simulink model "SerialSend"  (R2013a)
settings: Solver=ode45  StartTime=0.0  StopTime=inf  RelTol=1e-3
undefined symbols (not defined in the file or in its folder): none, Rec, SDTV, serial, videoinput
libraries: visionsinks x3, visionstatistics x2, imaqlib x2, instrumentlib x2, simulink x1, visionconversions x1, visiontextngfix x1, aerolibanimutils x1
settings Model: Creator=scastro  LastModifiedBy=sbiagion
settings OptimizationCC: ExpressionDepthLimit=2147483647  OptimizeModelRefInitCode=on  LifeSpan=1
settings DebuggingCC: StrictBusMsg=Warning
settings HardwareCC: ProdBitPerInt=16  ProdBitPerPointer=8  ProdIntDivRoundTo=Zero  ProdEndianess=LittleEndian  ProdWordSize=8  ProdHWDeviceType=Atmel->AVR
settings RTWCC: SystemTargetFile=realtime.tlc  GenerateMakefile=off  TemplateMakefile=realtime.tmf  Description=Real-Time Toolbox  RTWVerbose=off  ProcessScript=realtime_make_rtw_hook
settings CodeAppCC: IgnoreCustomStorageClasses=off  CustomSymbolStrType=$N$R$M  InternalIdentifier=Classic
settings STFCustomTargetCC: TargetLibSuffix=.a  GenerateSampleERTMain=on  CombineOutputUpdateFcns=on  ERTCustomFileBanners=on  SupportContinuousTime=off  SupportNonInlinedSFcns=off  MATLABClassNameForMDSCustomization=Simulink.SoftwareTarget.ERTCustomization  SystemTargetFile=realtime.tlc
settings ERTTargetCC: ParMdlRefBuildCompliant=off  CompOptLevelCompliant=off  ConcurrentExecutionCompliant=off  ERTFirstTimeCompliant=off  ModelStepFunctionPrototypeControlCompliant=off  CPPClassGenCompliant=off  ERTCustomFileTemplate=realtime_file_process.tlc

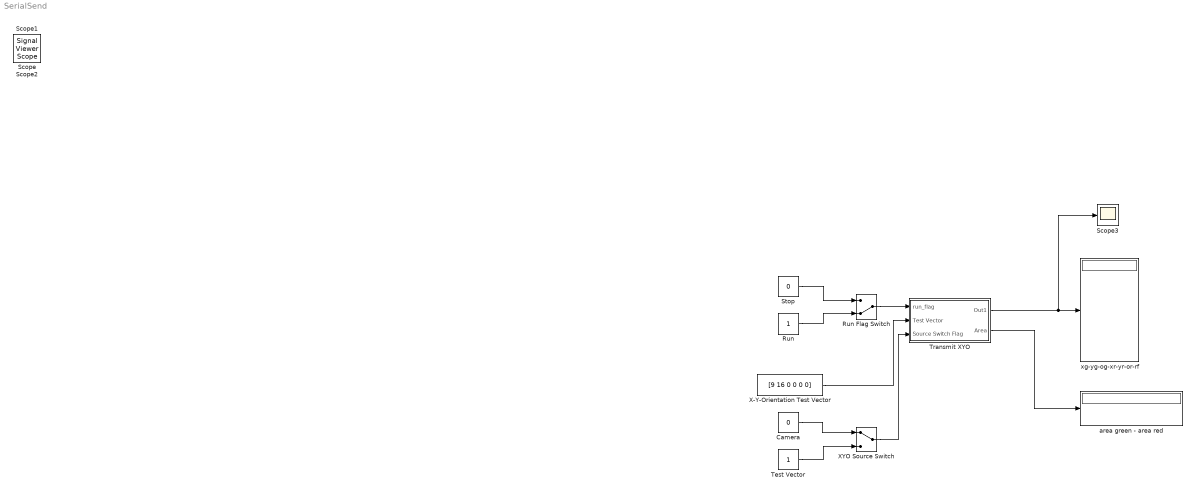
== system SerialSend ==
  Camera : Constant  Value=0  OutDataTypeStr=uint8
  Run : Constant  OutDataTypeStr=uint8
  Run Flag Switch : ManualSwitch  CurrentSetting=0
  Scope3 : Scope
      settings: ShowLegends=on  YMin=0  YMax=275
  Stop : Constant  Value=0  OutDataTypeStr=uint8
  Test Vector : Constant  OutDataTypeStr=uint8
  Transmit XYO : Subsystem
  X-Y-Orientation Test Vector : Constant  Value=[9 16 0 0 0 0]
  XYO Source Switch : ManualSwitch
  area green - area red : Display
  xg-yg-og-xr-yr-or-rf : Display
  Scope : SignalViewerScope  IOType=viewer  RefreshTime=0.035000
      settings: YMin=-40  YMax=70
  Scope1 : SignalViewerScope  IOType=viewer  ZoomMode=xonly  RefreshTime=0.035000
  Scope2 : SignalViewerScope  IOType=viewer  RefreshTime=0.035000
      settings: YMin=50  YMax=70  SaveName=ScopeData2
  wires:
  Run Flag Switch/1 -> Transmit XYO/1(run_flag)
  Stop/1 -> Run Flag Switch/1
  Run/1 -> Run Flag Switch/2
  Transmit XYO/1(Out1) -> Scope3/1, xg-yg-og-xr-yr-or-rf/1
  Camera/1 -> XYO Source Switch/1
  Test Vector/1 -> XYO Source Switch/2
  X-Y-Orientation Test Vector/1 -> Transmit XYO/2(Test Vector)
  XYO Source Switch/1 -> Transmit XYO/3(Source Switch Flag)
  Transmit XYO/2(Area) -> area green - area red/1

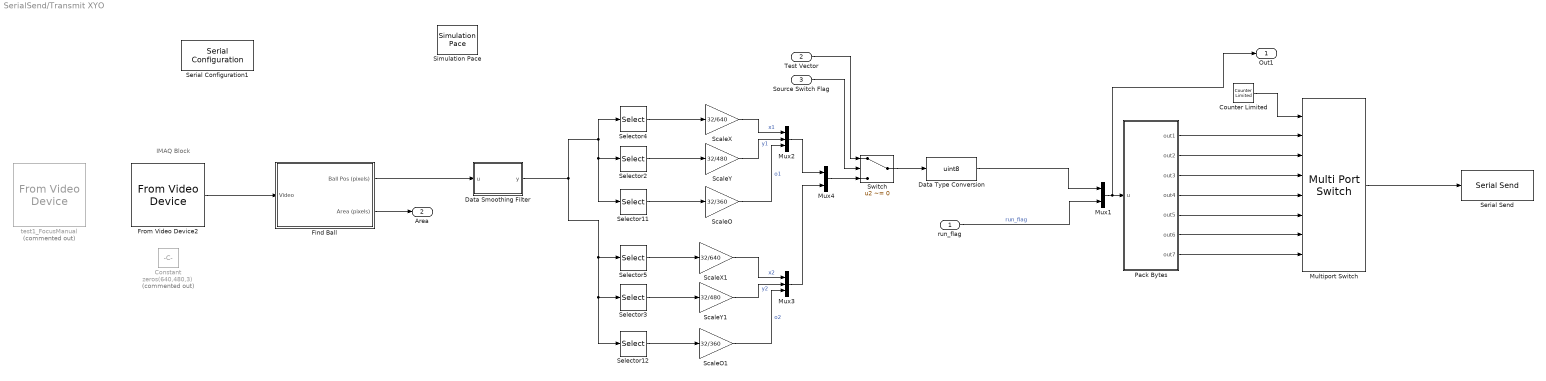
== system SerialSend/Transmit XYO ==
  note: IMAQ Block
  run_flag : Inport
  Test Vector : Inport  Port=2
  Source Switch Flag : Inport  Port=3
  Constant : Constant  Commented=on  Value=zeros(640,480,3)  SampleTime=0.1
  Counter Limited : simulink/Sources/Counter Limited  uplimit=6  tsamp=-1
  Data Smoothing Filter : MATLAB Function  TreatAsAtomicUnit=on
  Data Type Conversion : DataTypeConversion  OutDataTypeStr=uint8
  Find Ball : Subsystem
  From Video Device2 : imaqlib/From Video Device  DeviceMenu=winvideo 1 (Logitech Webcam Pro 9000)  Device=winvideo 1 (Logitech Webcam Pro 9000)  ObjConstructor=videoinput('winvideo', 1)  VideoFormatMenu=I420_640x480  VideoFormat=I420_640x480  VideoSource=input1  ROIPosition=[0 0 480 640]  EnableHWTrigger=off  TriggerConfiguration=none/none  SampleTime=0.1  OutputPortsMode=One multidimensional signal  DataType=double  CanDoHWTrigger=no  ReturnedColorSpace=rgb  BlockHandle=41.0012  ROIWidth=640  ROIHeight=480  ROIColumn=0  ROIRow=0  EngXMLPath=C:\Program Files\MATLAB\R2013a\toolbox\imaq\imaq\private  DevXMLPath=C:\Program Files\MATLAB\R2013a\toolbox\imaq\imaqadaptors\win64  EngLibPath=C:\Program Files\MATLAB\R2013a\toolbox\imaq\imaqblks\imaqmex\win64  ColorSpace=rgb  BayerSensorAlignment=grbg
  Multiport Switch : MultiPortSwitch  DataPortOrder=Zero-based contiguous  Inputs=7
  Mux1 : Mux  Inputs=2
  Mux2 : Mux  Inputs=3
  Mux3 : Mux  Inputs=3
  Mux4 : Mux  Inputs=2
  Pack Bytes : MATLAB Function  TreatAsAtomicUnit=on
  ScaleO : Gain  Gain=32/360
  ScaleO1 : Gain  Gain=32/360
  ScaleX : Gain  Gain=32/640
  ScaleX1 : Gain  Gain=32/640
  ScaleY : Gain  Gain=32/480
  ScaleY1 : Gain  Gain=32/480
  Selector11 : Selector  InputPortWidth=6  IndexOptions=Index vector (dialog)  Indices=3  OutputSizes=1
  Selector12 : Selector  InputPortWidth=6  IndexOptions=Index vector (dialog)  Indices=6  OutputSizes=1
  Selector2 : Selector  InputPortWidth=6  IndexOptions=Index vector (dialog)  Indices=2  OutputSizes=1
  Selector3 : Selector  InputPortWidth=6  IndexOptions=Index vector (dialog)  Indices=5  OutputSizes=1
  Selector4 : Selector  InputPortWidth=6  IndexOptions=Index vector (dialog)  Indices=1  OutputSizes=1
  Selector5 : Selector  InputPortWidth=6  IndexOptions=Index vector (dialog)  Indices=4  OutputSizes=1
  Serial Configuration1 : instrumentlib/Serial Configuration  Priority=-200000  ComPortMenu=<Please select a port...>  ComPort=COM4  ObjConstructor=serial('COM4');  BaudRate=9600  DataBits=8  Parity=none  StopBits=1  FlowControl=none  Timeout=10  ByteOrder=LittleEndian
  Serial Send : instrumentlib/Serial Send  ComPortMenu=<Please select a port...>  ComPort=COM4  ObjConstructor=serial('COM4');  Terminator=<none>  EnableBlockingMode=on
  Simulation Pace : aerolibanimutils/Simulation Pace  SimulationPace=1  SleepMode=MATLAB Thread  OutputPaceError=off  SampleTime=0.1
      settings: AttributesFormatString=%<SimulationPace> sec/sec
  Switch : Switch  Criteria=u2 ~= 0
  test1_FocusManual : imaqlib/From Video Device  Commented=on  DeviceMenu=winvideo 1 (Logitech Webcam Pro 9000)  Device=winvideo 1 (Logitech Webcam Pro 9000)  ObjConstructor=videoinput('winvideo', 1)  VideoFormatMenu=I420_640x480  VideoFormat=I420_640x480  VideoSource=input1  ROIPosition=[0 0 480 640]  EnableHWTrigger=off  TriggerConfiguration=none/none  SampleTime=0.1  OutputPortsMode=One multidimensional signal  DataType=double  CanDoHWTrigger=no  ReturnedColorSpace=rgb  BlockHandle=41.0012  ROIWidth=640  ROIHeight=480  ROIColumn=0  ROIRow=0  EngXMLPath=C:\Program Files\MATLAB\R2013a\toolbox\imaq\imaq\private  DevXMLPath=C:\Program Files\MATLAB\R2013a\toolbox\imaq\imaqadaptors\win64  EngLibPath=C:\Program Files\MATLAB\R2013a\toolbox\imaq\imaqblks\imaqmex\win64  ColorSpace=rgb  BayerSensorAlignment=grbg
  Out1 : Outport
  Area : Outport  Port=2
  wires:
  Find Ball/1(Ball Pos (pixels)) -> Data Smoothing Filter/1(u)
  Selector4/1 -> ScaleX/1
  Selector2/1 -> ScaleY/1
  ScaleX/1 -> Mux2/1  "x1"
  ScaleY/1 -> Mux2/2  "y1"
  Data Smoothing Filter/1(y) -> Selector12/1, Selector3/1, Selector5/1, Selector11/1, Selector2/1, Selector4/1
  Selector5/1 -> ScaleX1/1
  Selector3/1 -> ScaleY1/1
  ScaleX1/1 -> Mux3/1  "x2"
  ScaleY1/1 -> Mux3/2  "y2"
  Mux3/1 -> Mux4/2
  Mux4/1 -> Switch/3
  Counter Limited/1 -> Multiport Switch/1
  Mux2/1 -> Mux4/1
  ScaleO/1 -> Mux2/3  "o1"
  Selector12/1 -> ScaleO1/1
  ScaleO1/1 -> Mux3/3  "o2"
  Multiport Switch/1 -> Serial Send/1
  Pack Bytes/1(out1) -> Multiport Switch/2
  Pack Bytes/2(out2) -> Multiport Switch/3
  Pack Bytes/3(out3) -> Multiport Switch/4
  Pack Bytes/4(out4) -> Multiport Switch/5
  Pack Bytes/5(out5) -> Multiport Switch/6
  Pack Bytes/6(out6) -> Multiport Switch/7
  Selector11/1 -> ScaleO/1
  Mux1/1 -> Out1/1, Pack Bytes/1(u)
  Data Type Conversion/1 -> Mux1/1
  run_flag/1 -> Mux1/2  "run_flag"
  Pack Bytes/7(out7) -> Multiport Switch/8
  Test Vector/1 -> Switch/1
  Source Switch Flag/1 -> Switch/2
  Switch/1 -> Data Type Conversion/1
  From Video Device2/1 -> Find Ball/1(Video)
  Find Ball/2(Area (pixels)) -> Area/1

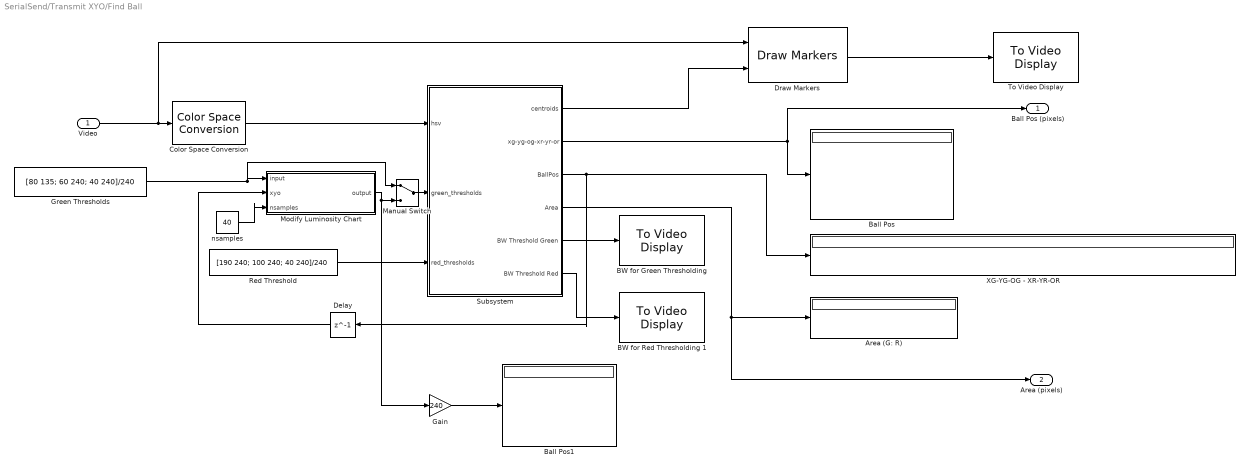
== system SerialSend/Transmit XYO/Find Ball ==
  Video : Inport
  Area (G: R) : Display
  "BW for Green Thresholding " : visionsinks/To Video Display  inputType=Obsolete  imagePorts=One multidimensional signal  OutputDevice=On-screen video monitor  fullScreen=off  videoWindowX=917  videoWindowY=30  saveWindowSize=off  videoWindowWidth=640  videoWindowHeight=480  dataOrg=Column-major  openAtMdlStart=on  isWindowOpen=on  inputColorFormat=RGB
  BW for Red Thresholding 1 : visionsinks/To Video Display  inputType=Obsolete  imagePorts=One multidimensional signal  OutputDevice=On-screen video monitor  fullScreen=off  videoWindowX=930  videoWindowY=402  saveWindowSize=off  videoWindowWidth=640  videoWindowHeight=480  dataOrg=Column-major  openAtMdlStart=on  isWindowOpen=on  inputColorFormat=RGB
  Ball Pos : Display
  Ball Pos1 : Display
  Color Space Conversion : visionconversions/Color Space  Conversion  conversion=Obsolete  conversionActive=R'G'B' to HSV  wp_str=D65  rec=Rec. 601 (SDTV)  sys=1125/60/2:1  imagePorts=One multidimensional signal
  Delay : Delay  DelayLength=1  InitialCondition=0
  Draw Markers : visiontextngfix/Draw Markers  shape=Circle  size=6  fill=off  fillClrSource=Specify via dialog  display=Black  intensity=200  color=[200 255 100]  opacity=0.6  viewport=Entire image  antialiasing=off  inType=Obsolete  imagePorts=One multidimensional signal  prodOutputMode=Binary point scaling  prodOutputWordLength=32  prodOutputFracLength=14  memoryMode=Specify word length  memoryWordLength=16  memoryFracLength=15  roundingMode=Floor  overflowMode=off
  Gain : Gain  Gain=240
  Green Thresholds : Constant  Value=[80 135; 60 240; 40 240]/240
  Manual Switch : ManualSwitch
  Modify Luminosity Chart : Stateflow chart  TreatAsAtomicUnit=on
  Red Threshold : Constant  Value=[190 240; 100 240; 40 240]/240
  Subsystem : Subsystem
  To Video Display : visionsinks/To Video Display  inputType=Obsolete  imagePorts=One multidimensional signal  OutputDevice=On-screen video monitor  fullScreen=off  videoWindowX=944  videoWindowY=-2  saveWindowSize=off  videoWindowWidth=640  videoWindowHeight=480  dataOrg=Column-major  openAtMdlStart=on  isWindowOpen=on  inputColorFormat=RGB
  XG-YG-OG - XR-YR-OR : Display
  nsamples : Constant  Value=40
  Ball Pos (pixels) : Outport
  Area (pixels) : Outport  Port=2
  wires:
  Draw Markers/1 -> To Video Display/1
  Video/1 -> Color Space Conversion/1, Draw Markers/1
  Subsystem/4(Area) -> Area (pixels)/1, Area (G: R)/1
  Color Space Conversion/1 -> Subsystem/1(hsv)
  Green Thresholds/1 -> Manual Switch/1, Modify Luminosity Chart/1(input)
  Red Threshold/1 -> Subsystem/3(red_thresholds)
  Subsystem/1(centroids) -> Draw Markers/2
  Subsystem/3(BallPos) -> Delay/1, XG-YG-OG - XR-YR-OR/1
  Subsystem/5(BW Threshold Green) -> "BW for Green Thresholding "/1
  Subsystem/6(BW Threshold Red) -> BW for Red Thresholding 1/1
  Subsystem/2(xg-yg-og-xr-yr-or) -> Ball Pos/1, Ball Pos (pixels)/1
  Modify Luminosity Chart/1(output) -> Manual Switch/2, Gain/1
  Delay/1 -> Modify Luminosity Chart/2(xyo)
  nsamples/1 -> Modify Luminosity Chart/3(nsamples)
  Manual Switch/1 -> Subsystem/2(green_thresholds)
  Gain/1 -> Ball Pos1/1

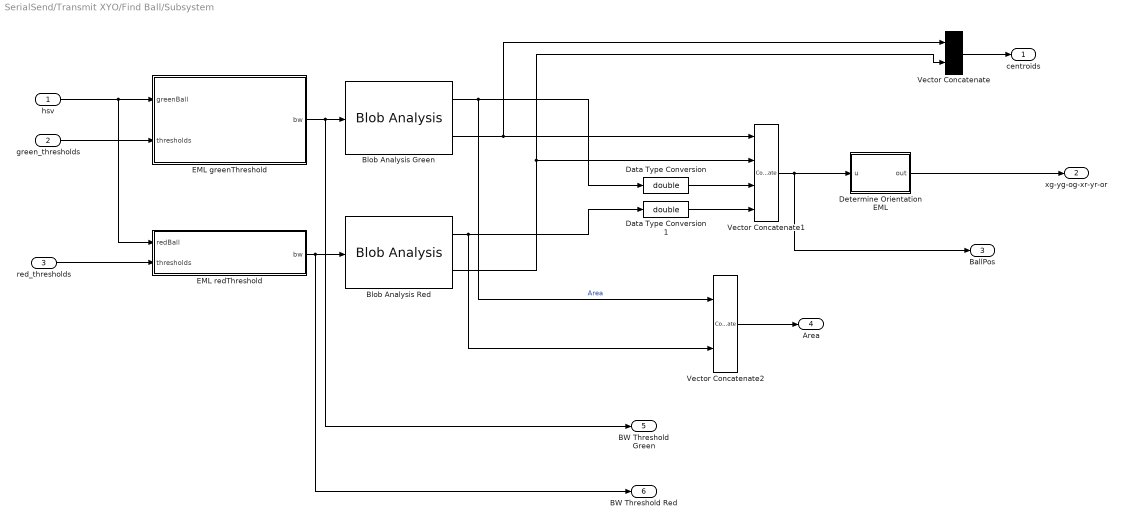
== system SerialSend/Transmit XYO/Find Ball/Subsystem ==
  hsv : Inport
  green_thresholds : Inport  Port=2
  red_thresholds : Inport  Port=3
  Blob Analysis Green : visionstatistics/Blob Analysis  Tag=vipblks_row_conv  area=on  centroid=on  bBox=off  majorAxis=off  minorAxis=off  angle=off  eccentricity=off  equivDiameterSq=off  extent=off  perimeter=off  maxBlobs=2  warnIfNumBlobsExceeded=off  isCount=off  useMinArea=on  minArea=50  useMaxArea=on  maxArea=1000  excludeBorderBlob=on  outDT=double  isOutVarDim=off  isFill=on  fillValues=-1  conn=8  isLabel=off  outputMode=Binary point scaling  outputWordLength=32  outputFracLength=16  firstCoeffMode=Binary point scaling  firstCoeffWordLength=16  firstCoeffFracLength=14  secondCoeffMode=Binary point scaling  secondCoeffWordLength=32  secondCoeffFracLength=16  accumMode=Binary point scaling  accumWordLength=32  accumFracLength=0  prodOutputMode=Binary point scaling  prodOutputWordLength=32  prodOutputFracLength=16  roundingMode=Floor  overflowMode=off
  Blob Analysis Red : visionstatistics/Blob Analysis  Tag=vipblks_row_conv  area=on  centroid=on  bBox=off  majorAxis=off  minorAxis=off  angle=off  eccentricity=off  equivDiameterSq=off  extent=off  perimeter=off  maxBlobs=2  warnIfNumBlobsExceeded=off  isCount=off  useMinArea=on  minArea=80  useMaxArea=on  maxArea=2000  excludeBorderBlob=on  outDT=double  isOutVarDim=off  isFill=on  fillValues=-1  conn=8  isLabel=off  outputMode=Binary point scaling  outputWordLength=32  outputFracLength=16  firstCoeffMode=Binary point scaling  firstCoeffWordLength=16  firstCoeffFracLength=14  secondCoeffMode=Binary point scaling  secondCoeffWordLength=32  secondCoeffFracLength=16  accumMode=Binary point scaling  accumWordLength=32  accumFracLength=0  prodOutputMode=Binary point scaling  prodOutputWordLength=32  prodOutputFracLength=16  roundingMode=Floor  overflowMode=off
  Data Type Conversion : DataTypeConversion  OutDataTypeStr=double
  Data Type Conversion1 : DataTypeConversion  OutDataTypeStr=double
  Determine Orientation EML : MATLAB Function  TreatAsAtomicUnit=on
  EML greenThreshold : MATLAB Function  TreatAsAtomicUnit=on
  EML redThreshold : MATLAB Function  TreatAsAtomicUnit=on
  Vector Concatenate : Concatenate  Mode=Multidimensional array
  Vector Concatenate1 : Concatenate  NumInputs=4  Mode=Multidimensional array  ConcatenateDimension=2
  Vector Concatenate2 : Concatenate  Mode=Multidimensional array  ConcatenateDimension=2
  centroids : Outport
  xg-yg-og-xr-yr-or : Outport  Port=2
  BallPos : Outport  Port=3
  Area : Outport  Port=4
  BW Threshold Green : Outport  Port=5
  BW Threshold Red : Outport  Port=6
  wires:
  Data Type Conversion/1 -> Vector Concatenate1/3
  green_thresholds/1 -> EML greenThreshold/2(thresholds)
  Data Type Conversion1/1 -> Vector Concatenate1/4
  EML redThreshold/1(bw) -> BW Threshold Red/1, Blob Analysis Red/1
  EML greenThreshold/1(bw) -> BW Threshold Green/1, Blob Analysis Green/1
  Vector Concatenate2/1 -> Area/1
  Blob Analysis Red/1 -> Data Type Conversion1/1, Vector Concatenate2/2
  Blob Analysis Green/1 -> Data Type Conversion/1, Vector Concatenate2/1  "Area"
  red_thresholds/1 -> EML redThreshold/2(thresholds)
  hsv/1 -> EML redThreshold/1(redBall), EML greenThreshold/1(greenBall)
  Blob Analysis Red/2 -> Vector Concatenate/2, Vector Concatenate1/2
  Blob Analysis Green/2 -> Vector Concatenate/1, Vector Concatenate1/1
  Vector Concatenate/1 -> centroids/1
  Vector Concatenate1/1 -> BallPos/1, Determine Orientation EML/1(u)
  Determine Orientation EML/1(out) -> xg-yg-og-xr-yr-or/1

== matlab function SerialSend/Transmit XYO/Data Smoothing Filter ==
  data: u input; y output
function y = fcn(u)
%#codegen
n = 1; % number of points to sample
persistent x1temp x2temp y1temp y2temp o1temp o2temp ii
if isempty(x1temp)
    x1temp = zeros(1,n);
end
if isempty(x2temp)
    x2temp = zeros(1,n);
end
if isempty(y1temp)
    y1temp = zeros(1,n);
end
if isempty(y2temp)
    y2temp = zeros(1,n);
end
if isempty(o1temp)
    o1temp = zeros(1,n);
end
if isempty(o2temp)
    o2temp = zeros(1,n);
end
if isempty(ii)
    ii = 1;
end
if ii == (n+1)
    ii = 1;
end

x1temp(ii) = u(1);
y1temp(ii) = u(2);
o1temp(ii) = u(3);
x2temp(ii) = u(4);
y2temp(ii) = u(5);
o2temp(ii) = u(6);

ii = ii+1;

y = zeros(1,6);
y(1) = mean(x1temp);
y(2) = mean(y1temp);
y(3) = mean(o1temp);
y(4) = mean(x2temp);
y(5) = mean(y2temp);
y(6) = mean(o2temp);

== matlab function SerialSend/Transmit XYO/Find Ball/Subsystem/EML greenThreshold ==
  data: greenBall input; bw output; thresholds input size=[3 2]
function bw = greenThreshold(greenBall,thresholds)
% This block supports the Embedded MATLAB subset.
% See the help menu for details. 
ht = thresholds(1,1:2);
st = thresholds(2,1:2);
lt = thresholds(3,1:2);

%% Extract each color
% Next we using indexing to extract three 2D matrices from the 3D image
% data corresponding to the red, green, and blue components of the image.
h = greenBall(:,:,1);
s = greenBall(:,:,2);
l = greenBall(:,:,3);

%% Threshold the image
% Now we can set a threshold to separate the parts of the image that we
% consider to be green from the rest.
% 78 92
% bw = (h >= 78/240) & (h <= 125/240) & (s >= 100/240);
% % bw = s <= 40/240; % for center of green led's
% bw = s <= 200/240;
% bw = s >= 80/240;
% bw = (s >= 80/240) & (s <= 200/240);
% bw = h >= 80/240;
% bw = h <= 150/240;
% bw = (h >= 90/240) & (h <= 130/240) & (s >= 90/240) & (s <= 200);
bw = (h >= ht(1)) & (h <= ht(2)) & (s >= st(1)) & (s <= st(2)) & (l >= lt(1)) & (l <= lt(2));

== matlab function SerialSend/Transmit XYO/Pack Bytes ==
  data: u input uint8 size=7; out1 output uint8 size=1; out2 output uint8 size=1; out3 output uint8 size=1; out4 output; out5 output; out6 output; out7 output
function [out1, out2, out3, out4, out5, out6, out7] = fcn(u)
%#codegen

% test vector
% u = uint8([2 7 1 3 5 2]);

% pack x1 data for packet 1
x1 = u(1);
x1shifted = bitshift(x1,3);
id = 0;
out1 = id+x1shifted;

% pack y1 data for packet 2
y1 = u(2);
y1shifted = bitshift(y1,3);
id = 1;
out2 = id+y1shifted;

% pack o1 data for packet 3
o1 = u(3);
o1shifted = bitshift(o1,3);
id = 2;
out3 = id+o1shifted;

% pack x2 data for packet 4
x2 = u(4);
x2shifted = bitshift(x2,3);
id = 3;
out4 = id+x2shifted;

% pack y2 data for packet 5
y2 = u(5);
y2shifted = bitshift(y2,3);
id = 4;
out5 = id+y2shifted;

% pack o2 data for packet 6
o2 = u(6);
o2shifted = bitshift(o2,3);
id = 5;
out6 = id+o2shifted;

% pack run flag
rf = u(7);
rfshifted = bitshift(rf,3);
id = 6;
out7 = id+rfshifted;

== stateflow chart SerialSend/Transmit XYO/Find Ball/Modify Luminosity Chart ==
  state lowluminosity
    during:
    [val i] = find(xyo(1:2,1:2) == -1);
    if ~isempty(i)
    counter = counter + 1; % could not find a coordinate
    else
    counter = 0;
    end
    temp = input;
    temp(3,1) = 40/240;
    output = temp;
  state highluminosity
    during:
    [val i] = find(xyo(1:2,1:2) == -1);
    if ~isempty(i)
    counter = counter + 1; % could not find a coordinate
    else
    counter = 0;
    end
    temp = input;
    temp(3,1) = 55/240;
    output = temp;
  (default) -> lowluminosity : {counter = 0;}
  lowluminosity -> highluminosity : [counter > nsamples] {counter = 0;}
  highluminosity -> lowluminosity : [counter > nsamples] {counter = 0;}
  data: input input; output output; xyo input; counter local; val local size=8; i local size=8; temp local; nsamples input

== matlab function SerialSend/Transmit XYO/Find Ball/Subsystem/EML redThreshold ==
  data: redBall input; bw output; thresholds input size=[3 2]
function bw = redThreshold(redBall,thresholds)
% This block supports the Embedded MATLAB subset.
% See the help menu for details. 
ht = thresholds(1,1:2);
st = thresholds(2,1:2);
lt = thresholds(3,1:2);

%% Extract each color
% Next we using indexing to extract three 2D matrices from the 3D image
% data corresponding to the red, green, and blue components of the image.
h = redBall(:,:,1);
s = redBall(:,:,2);
l = redBall(:,:,3);

%% Threshold the image
% Now we can set a threshold to separate the parts of the image that we
% consider to be green from the rest.
% 220 worked very well
% bw = (h > 220/240) & (s >= 100/240);
% bw = s >= 120/240;  
% bw = (h >= ht(1)) & (h <= ht(2));
% bw = (s >= st(1)) & (s <= st(2));
% bw = (((h >= 0) & (h <= 3))|((h >= ht(1)) & (h <= ht(2)))) & (s >= st(1)) & (s <= st(2)) & (l >= lt(1)) & (l <= lt(2));
bw = ((h >= ht(1)) & (h <= ht(2))) & (s >= st(1)) & (s <= st(2)) & (l >= lt(1)) & (l <= lt(2));
% bw = (h > 220/240) & (s >= 100/240);

== matlab function SerialSend/Transmit XYO/Find Ball/Subsystem/Determine Orientation EML ==
  data: u input size=[2 6]; out output
function out = fcn(u)
%#codegen

% extract all variables
xgv = u(:,1);
ygv = u(:,2);
xrv = u(:,3);
yrv = u(:,4);
agv = u(:,5);
arv = u(:,6);

% transform axis such that x = 0, y = 0 is located at bottom left of screen
ygv = 480-ygv; 
yrv = 480-yrv;

% create frindex, brindex, fgindex, bgindex
[~, bgindex] = max(agv);
[~, brindex] = max(arv);

if bgindex == 1
    fgindex = 2;
else
    fgindex = 1;
end

if brindex == 1
    frindex = 2;
else
    frindex = 1;
end

fg = [xgv(fgindex) ygv(fgindex)]; % [x y] coordinates for front of green
bg = [xgv(bgindex) ygv(bgindex)]; % [x y] coordinates for back of green
fr = [xrv(frindex) yrv(frindex)]; % [x y] coordinates for front of red
br = [xrv(brindex) yrv(brindex)]; % [x y] coordinates for back of red

% determine orientation
og = atan2(fg(2)-bg(2),fg(1)-bg(1))*180/pi;
og  = mod(og+360,360);
or = atan2(fr(2)-br(2),fr(1)-br(1))*180/pi;
or = mod(or+360,360);

% determine xr, yr, or, xg, yg, og
xg = mean([fg(1) bg(1)]);
yg = mean([fg(2) bg(2)]);
xr = mean([fr(1) br(1)]);
yr = mean([fr(2) br(2)]);

out = [xg yg og xr yr or];
